simulink model "Traffic_Led"  (R2024b)
settings: Solver=VariableStepAuto  StartTime=0.0  StopTime=10.0  RelTol=1e-3
settings Model: Creator=Ahmad  LastModifiedBy=Ahmad

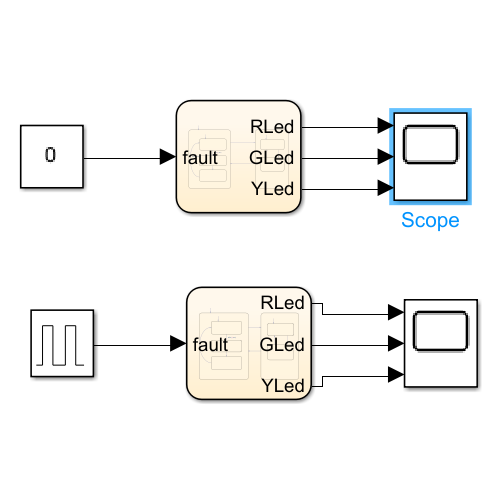
[thumbnail: Simulink's stored preview of the top-level diagram]
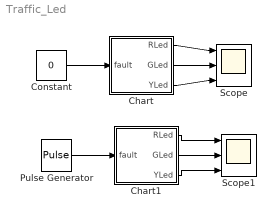
== system Traffic_Led ==
  Chart : Stateflow chart  TreatAsAtomicUnit=on
  Chart1 : Stateflow chart  TreatAsAtomicUnit=on
  Constant : Constant  Value=0
  Pulse Generator : DiscretePulseGenerator  PulseType=Time based  Period=10  PulseWidth=50
  Scope : Scope  NumInputPorts=3
  Scope1 : Scope  NumInputPorts=3
  wires:
  Constant/1 -> Chart/1(fault)
  Chart/1(RLed) -> Scope/1
  Chart/2(GLed) -> Scope/2
  Chart/3(YLed) -> Scope/3
  Chart1/1(RLed) -> Scope1/1
  Chart1/2(GLed) -> Scope1/2
  Chart1/3(YLed) -> Scope1/3
  Pulse Generator/1 -> Chart1/1(fault)

== stateflow chart Traffic_Led/Chart1 ==
  state NormalMode
    state Stop
      entry:
      RLed=1;
      exit:
      RLed=0;
    note: after ( 1 , sec )
    state Go
      entry:
      GLed=1;
      exit:
      GLed=0;
    state PTS
      entry:
      YLed=1;
      exit:
      YLed=0;
    (default) -> Stop
    PTS -> Stop : after(1,sec)
    Stop -> Go
    Go -> PTS : after(1,sec)
  state FaultMode
    state ON
      entry:
      RLed=1;
    state OFF
      entry:
      RLed=0;
    (default) -> ON
    OFF -> ON : after(1,sec)
    ON -> OFF : after(1,sec)
  (default) -> NormalMode
  NormalMode -> FaultMode : [fault==1]
  FaultMode -> NormalMode : [fault==0]
  data: fault input; RLed output; GLed output; YLed output

== stateflow chart Traffic_Led/Chart ==
  state NormalMode
    state Stop
      entry:
      RLed=1;
      exit:
      RLed=0;
    note: after ( 1 , sec )
    note: after ( 1 , sec )
    state Go
      entry:
      GLed=1;
      exit:
      GLed=0;
    state PTS
      entry:
      YLed=1;
      exit:
      YLed=0;
    (default) -> Stop
    PTS -> Stop
    Stop -> Go
    Go -> PTS : after(1,sec)
  state FaultMode
    state ON
      entry:
      RLed=1;
    state OFF
      entry:
      RLed=0;
    (default) -> ON
    OFF -> ON : after(1,sec)
    ON -> OFF : after(1,sec)
  (default) -> NormalMode
  NormalMode -> FaultMode : [fault==1]
  FaultMode -> NormalMode : [fault==0]
  data: fault input; RLed output; GLed output; YLed output
